simulink model "Full_Observer_Based_Controller"  (R2020b)
settings: Solver=VariableStepAuto  StartTime=0.0  StopTime=5  RelTol=1e-3
undefined symbols (not defined in the file): A, B, C, D, L
settings Model: Creator=Alvaro  LastModifiedBy=Alvaro

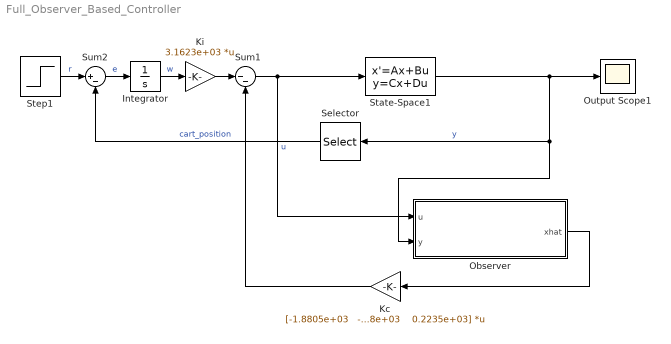
== system Full_Observer_Based_Controller ==
  Integrator : Integrator
  Kc : Gain  Gain="[-1.8805e+03   -0.5277e+03    1.1078e+03    0.2235e+03]"  Multiplication=Matrix(K*u)
  Ki : Gain  Gain=3.1623e+03  Multiplication=Matrix(K*u)
  Observer : Subsystem  mask(Full Order Luenberger Observer){A=A, B=B, C=C, D=D}
      mask prompts: A "State Matrix (A)"; B "Input Matrix (B)"; C "Ouput Matrix (C)"; D "Feedforward Matrix (D)"
      mask help:
      | Continuous Luenberger Observer Block.
      | It will estimate all the states of a given observable open-loop system.
      mask Display: disp('Full Order \n Luenberger Observer')
  Output Scope1 : Scope
  Selector : Selector  InputPortWidth=2  IndexOptions=Index vector (dialog)  Indices=[1]  OutputSizes=1
  State-Space1 : StateSpace  A=A  B=B  C=[1 0 0 0; 0 0 1 0]  D=[0; 0]  InitialCondition=0
  Step1 : Step  Time=0.01  After=0.2  SampleTime=0
  Sum1 : Sum  Inputs=|--
  Sum2 : Sum  Inputs=|+-
  wires:
  Observer/1(xhat) -> Kc/1
  Selector/1 -> Sum2/2  "cart_position"
  Ki/1 -> Sum1/1
  State-Space1/1 -> Output Scope1/1, Selector/1, Observer/2(y)  "y"
  Step1/1 -> Sum2/1  "r"
  Kc/1 -> Sum1/2
  Integrator/1 -> Ki/1  "w"
  Sum1/1 -> Observer/1(u), State-Space1/1  "u"
  Sum2/1 -> Integrator/1  "e"

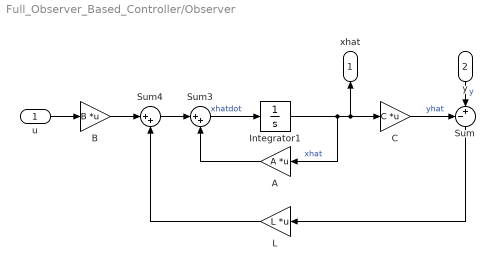
== system Full_Observer_Based_Controller/Observer ==
  u : Inport
  y : Inport  Port=2
  A : Gain  Gain=A  Multiplication=Matrix(K*u)
  B : Gain  Gain=B  Multiplication=Matrix(K*u)
  C : Gain  Gain=C  Multiplication=Matrix(K*u)
  Integrator1 : Integrator
  L : Gain  Gain=L  Multiplication=Matrix(K*u)
  Sum : Sum  Inputs=-+|
  Sum3 : Sum  Inputs=|++
  Sum4 : Sum  Inputs=|++
  xhat : Outport
  wires:
  A/1 -> Sum3/2
  Sum3/1 -> Integrator1/1  "xhatdot"
  Integrator1/1 -> xhat/1, C/1, A/1  "xhat"
  y/1 -> Sum/2  "y"
  Sum4/1 -> Sum3/1
  C/1 -> Sum/1  "yhat"
  Sum/1 -> L/1
  L/1 -> Sum4/2
  B/1 -> Sum4/1
  u/1 -> B/1
